simulink model "Halleffect"  (R2024b)
settings: Solver=FixedStepAuto  StartTime=0.0  StopTime=13  FixedStep=0.01  RelTol=1e-3  EnableMultiTasking=on
libraries: stm32f4xxblockslib x1
settings Model: STM32="{\"AnalogInput\":{\"ID\":\"untitled:1\"}}"  PacingRate=10  Creator=ASUS  LastModifiedBy=ASUS
settings OptimizationCC: DefaultParameterBehavior=Inlined  EnhancedBackFolding=on  PassReuseOutputArgsAs=Individual arguments  ZeroExternalMemoryAtStartup=off  ZeroInternalMemoryAtStartup=off  MaxStackSize=512  OptimizeBlockOrder=speed  DifferentSizesBufferReuse=on  OptimizationCustomize=off  EfficientTunableParamExpr=on
settings DebuggingCC: ParameterTunabilityLossMsg=error
settings HardwareCC: ProdBitPerPointer=32  ProdBitPerSizeT=32  ProdBitPerPtrDiffT=32  ProdLargestAtomicInteger=Long  ProdLargestAtomicFloat=Double  ProdWordSize=32  ProdLongLongMode=on  ProdHWDeviceType=ARM Compatible->ARM Cortex-M
settings SFSimCC: MATLABDynamicMemAlloc=off
settings RTWCC: Description=Embedded Coder  SystemTargetFile=ert.tlc  HardwareBoard=STM32G4xx Based  TemplateMakefile=ert_default_tmf  Toolchain=GNU Tools for ARM Embedded Processors
settings CodeAppCC: ForceParamTrailComments=on  IgnoreCustomStorageClasses=off  OperatorAnnotations=on  SimulinkDataObjDesc=on  SFDataObjDesc=on  InsertBlockDesc=on
settings ERTTargetCC: TargetLangStandard=C99 (ISO)  CodeReplacementLibrary=ARM Cortex-M  ExtModeTransport=3  ExtModeStaticAlloc=on  ExtModeStaticAllocSize=2048  ExtModeMexFile=ext_xcp  ExtModeIntrfLevel=Level2 - Open

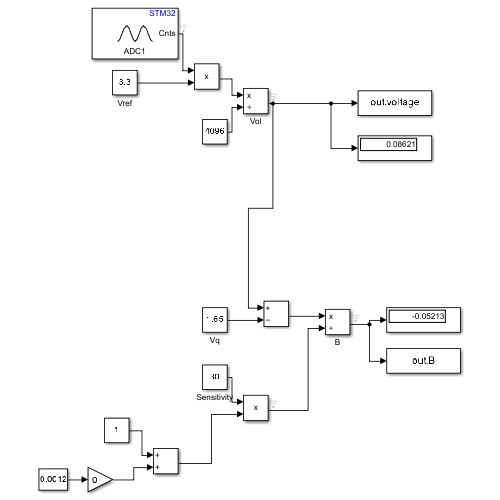
[thumbnail: Simulink's stored preview of the top-level diagram]
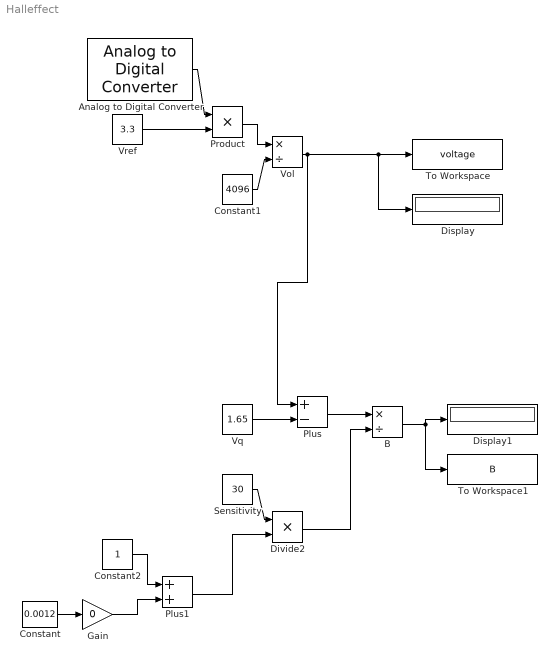
== system Halleffect ==
  Analog to Digital Converter : stm32f4xxblockslib/Analog to Digital Converter  ADCModule=ADC1  ConversionGroup=Regular  TriggerMode=Trigger and read  NumberOfConversions=1  EnableBufferConv=off  BufferLength=1  OutputStatus=off  SampleTime=-1  EnableSimPort=off  hoistedMaskSrc=ECSoC/ECSimCodegen/Analog to Digital Converter
  B : Product  Inputs=*/
  Constant : Constant  Value=0.0012
  Constant1 : Constant  Value=4096
  Constant2 : Constant
  Display : Display
  Display1 : Display
  Divide2 : Product  Inputs=**
  Gain : Gain  Gain=0
  Plus : Sum  Inputs=+-
  Plus1 : Sum
  Product : Product
  Sensitivity : Constant  Value=30
  To Workspace : ToWorkspace  VariableName=voltage  SaveFormat=Structure With Time  SampleTime=-1
  To Workspace1 : ToWorkspace  VariableName=B  SaveFormat=Structure With Time  SampleTime=-1
  Vol : Product  Inputs=*/
  Vq : Constant  Value=1.65
  Vref : Constant  Value=3.3
  wires:
  Analog to Digital Converter/1 -> Product/1
  Vref/1 -> Product/2
  Product/1 -> Vol/1
  Constant1/1 -> Vol/2
  Vol/1 -> To Workspace/1, Display/1, Plus/1
  Vq/1 -> Plus/2
  Plus/1 -> B/1
  Sensitivity/1 -> Divide2/1
  Constant2/1 -> Plus1/1
  Constant/1 -> Gain/1
  Gain/1 -> Plus1/2
  Plus1/1 -> Divide2/2
  Divide2/1 -> B/2
  B/1 -> To Workspace1/1, Display1/1
